simulink model "planta"  (Simulink 7.3)
settings: Solver=ode45  StartTime=0.0  StopTime=900  MaxStep=0.03  MinStep=0.01  RelTol=1e-3
settings Model: Creator=Daniel  LastModifiedBy=Daniel
settings SolverCC: InitialStep=0.01

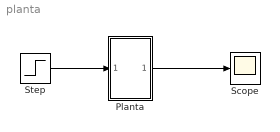
== system planta ==
  Planta : Subsystem
  Scope : Scope
      settings: DataFormat=Array
  Step : Step  Time=5  After=50  SampleTime=0
  wires:
  Step/1 -> Planta/1(In1)
  Planta/1(Out1) -> Scope/1

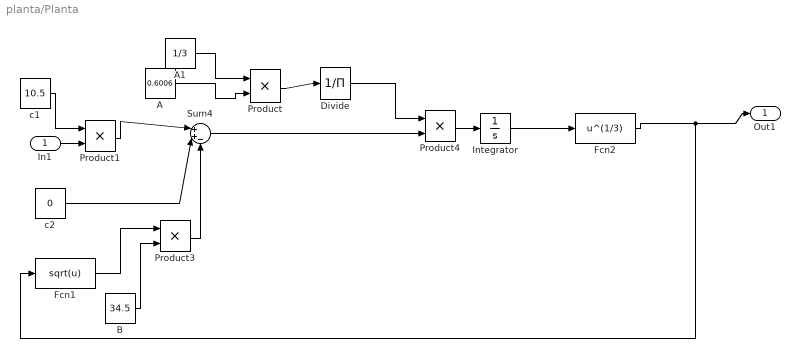
== system planta/Planta ==
  In1 : Inport
  A : Constant  Value=0.6006  OutDataType=fixdt(1, 16)  OutScaling=2^0
  A1 : Constant  Value=1/3  OutDataType=fixdt(1, 16)  OutScaling=2^0
  B : Constant  Value=34.5  OutDataType=fixdt(1, 16)  OutScaling=2^0
  Divide : Product  Inputs=/  OutDataType=fixdt(1, 16)  OutScaling=2^-10
  Fcn1 : Fcn  Expr=sqrt(u)  SampleTime=0.1
  Fcn2 : Fcn  Expr=u^(1/3)  SampleTime=0.1
  Integrator : Integrator  InitialCondition=1  LimitOutput=on  UpperSaturationLimit=70  LowerSaturationLimit=0.1
  Product : Product  Inputs=**  OutDataType=fixdt(1, 16)  OutScaling=2^0  RndMeth=Zero
  Product1 : Product  OutDataType=fixdt(1, 16)  OutScaling=2^0  SampleTime=0.1  RndMeth=Zero
  Product3 : Product  OutDataType=fixdt(1, 16)  OutScaling=2^0  SampleTime=0.1  RndMeth=Zero
  Product4 : Product  OutDataType=fixdt(1, 16)  OutScaling=2^0  SampleTime=0.1  RndMeth=Zero
  Sum4 : Sum  Inputs=|++-  OutDataType=fixdt(1, 16)  OutScaling=2^0
  c1 : Constant  Value=10.5  OutDataType=fixdt(1, 16)  OutScaling=2^0
  c2 : Constant  Value=0  OutDataType=fixdt(1, 16)  OutScaling=2^0
  Out1 : Outport
  wires:
  c1/1 -> Product1/1
  Product1/1 -> Sum4/1
  c2/1 -> Sum4/2
  Fcn1/1 -> Product3/1
  B/1 -> Product3/2
  Product3/1 -> Sum4/3
  Sum4/1 -> Product4/2
  Divide/1 -> Product4/1
  Product/1 -> Divide/1
  Product4/1 -> Integrator/1
  In1/1 -> Product1/2
  A/1 -> Product/2
  A1/1 -> Product/1
  Integrator/1 -> Fcn2/1
  Fcn2/1 -> Fcn1/1, Out1/1
